simulink model "Test_Euler2DCM2"  (Simulink 7.5)
settings: Solver=FixedStepDiscrete  StartTime=0.0  StopTime=1  RelTol=1e-3
values from neighbouring files (symbols this model uses):
  apSampleTime = 0.01    [demoz2SlugsV5.m]
libraries: aerolibutil x1
settings Model: Creator=Robert  LastModifiedBy=Robert

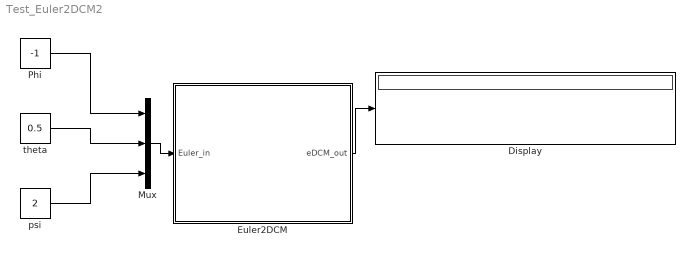
== system Test_Euler2DCM2 ==
  Display : Display
  Euler2DCM : Subsystem
  Mux : Mux  Inputs=3
  Phi : Constant  Value=-1  OutDataTypeMode=single  OutDataType=fixdt(1, 16)  OutScaling=2^0  OutDataTypeStr=single
  psi : Constant  Value=2  OutDataTypeMode=single  OutDataType=fixdt(1, 16)  OutScaling=2^0  OutDataTypeStr=single
  theta : Constant  Value=0.5  OutDataTypeMode=single  OutDataType=fixdt(1, 16)  OutScaling=2^0  OutDataTypeStr=single
  wires:
  Phi/1 -> Mux/1
  theta/1 -> Mux/2
  psi/1 -> Mux/3
  Euler2DCM/1(eDCM_out) -> Display/1
  Mux/1 -> Euler2DCM/1(Euler_in)

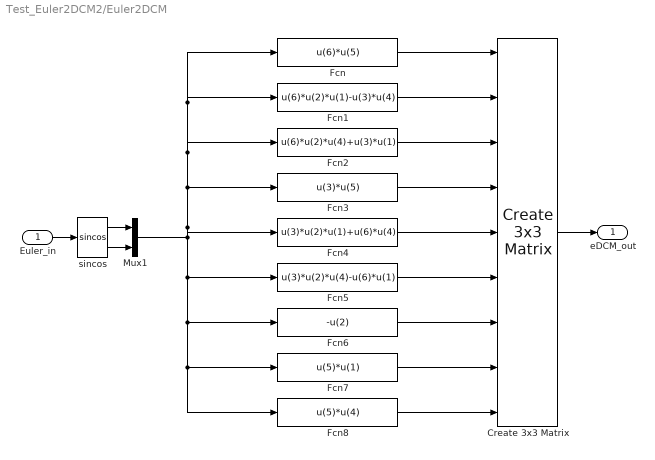
== system Test_Euler2DCM2/Euler2DCM ==
  Euler_in : Inport  PortDimensions=3
  Create 3x3 Matrix : aerolibutil/Create 3x3 Matrix  SystemSampleTime=-1
  Fcn : Fcn  Expr=u(6)*u(5)  SampleTime=apSampleTime
  Fcn1 : Fcn  Expr=u(6)*u(2)*u(1)-u(3)*u(4)  SampleTime=apSampleTime
  Fcn2 : Fcn  Expr=u(6)*u(2)*u(4)+u(3)*u(1)  SampleTime=apSampleTime
  Fcn3 : Fcn  Expr=u(3)*u(5)  SampleTime=apSampleTime
  Fcn4 : Fcn  Expr=u(3)*u(2)*u(1)+u(6)*u(4)  SampleTime=apSampleTime
  Fcn5 : Fcn  Expr=u(3)*u(2)*u(4)-u(6)*u(1)  SampleTime=apSampleTime
  Fcn6 : Fcn  Expr=-u(2)  SampleTime=apSampleTime
  Fcn7 : Fcn  Expr=u(5)*u(1)  SampleTime=apSampleTime
  Fcn8 : Fcn  Expr=u(5)*u(4)  SampleTime=apSampleTime
  Mux1 : Mux  Inputs=2
  sincos : Trigonometry  Operator=sincos
  eDCM_out : Outport  PortDimensions=[3,3]
  wires:
  Euler_in/1 -> sincos/1
  sincos/1 -> Mux1/1
  sincos/2 -> Mux1/2
  Create 3x3 Matrix/1 -> eDCM_out/1
  Mux1/1 -> Fcn/1, Fcn1/1, Fcn2/1, Fcn3/1, Fcn4/1, Fcn5/1, Fcn8/1, Fcn7/1, Fcn6/1
  Fcn/1 -> Create 3x3 Matrix/1
  Fcn1/1 -> Create 3x3 Matrix/2
  Fcn2/1 -> Create 3x3 Matrix/3
  Fcn3/1 -> Create 3x3 Matrix/4
  Fcn4/1 -> Create 3x3 Matrix/5
  Fcn5/1 -> Create 3x3 Matrix/6
  Fcn6/1 -> Create 3x3 Matrix/7
  Fcn7/1 -> Create 3x3 Matrix/8
  Fcn8/1 -> Create 3x3 Matrix/9
